simulink model "NSFsim_syn_2023"  (R2020b)
settings: Solver=FixedStepAuto  StartTime=0.0  StopTime=10  FixedStep=tstep  RelTol=1e-3
model workspace (MAT data in the model file):
  GSorder = 3
  TargetTime = 1
  blankingDur = 0.012
  mwavedur = 0.01
  rngseed = 1000
  stimfreq = 20
  tstep = 0.0001
  wc = 0.6
libraries: dspstat3 x4
settings Model: OrderedModelArguments=off  Creator=akif  LastModifiedBy=akif
settings SolverCC: AlgebraicLoopSolver=LineSearch
settings DebuggingCC: ArithmeticOperatorsInVariantConditions=warning
settings SFSimCC: CustomCodeUndefinedFunction=UseInterfaceOnly

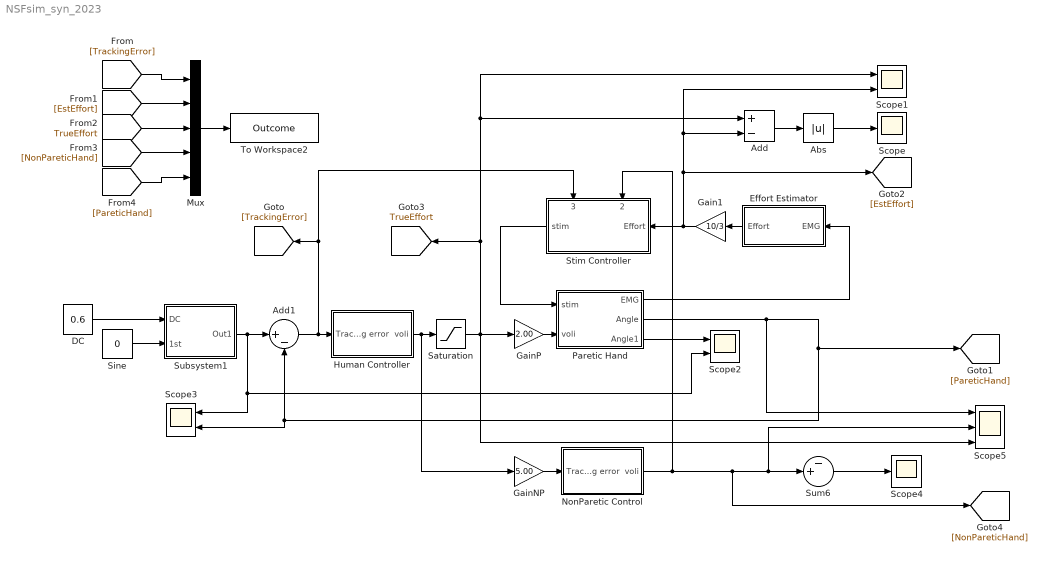
== system NSFsim_syn_2023 ==
  Abs : Abs
  Add : Sum  Inputs=+-
  Add1 : Sum  Inputs=|+-  InputSameDT=on  AccumDataTypeStr=double  OutDataTypeStr=Inherit: Inherit via back propagation
  DC : Constant  Value=0.6
  Effort Estimator : Subsystem
  Gain1 : Gain  Gain=10/3
  GainNP : Gain  Gain=5.00
  GainP : Gain  Gain=2.00
  Human Controller : Subsystem
  Mux : Mux  Inputs=5
  NonParetic Control : Subsystem
  Paretic Hand : Subsystem
  Saturation : Saturate  UpperLimit=0.3  LowerLimit=0
  Scope : Scope
  Scope1 : Scope  NumInputPorts=2
  Scope2 : Scope  NumInputPorts=2
  Scope3 : Scope  NumInputPorts=2
  Scope4 : Scope
  Scope5 : Scope  NumInputPorts=3
  Sine : Constant  Value=0
  Stim Controller : Subsystem
      settings: PortSchema="{\"entries\":[{\"content\":{\"sides\":[{\"content\":{\"connectorIds\":[\"In1\"]},\"type\":\"ConnectorPlacement.EquallySpacedRectSide\",\"uuid\":\"20982ba9-d3c9-405a-8644-0483e80e19b0\"},{\"content\":{\"connectorIds\":[\"Out1\"],\"side\":\"RIGHT\"},\"type\":\"ConnectorPlacement.EquallySpacedRectSide\",\"uuid\":\"dfaac367-100c-4435-9839-729069c8d6e0\"},{\"content\":{\"connectorIds\":[\"In2\",\"In3\"],\"side\":\"TOP\"},\"type\":\"ConnectorPlacement.EquallySpacedRectSide\",\"uuid\":\"458cbc31-cb02-49e5-bc75-9e60cc365810\"},{\"content\":{\"connectorIds\":[],\"side\":\"BOTTOM\"},\"type\":\"ConnectorPlacement.EquallySpacedRectSide\",\"uuid\":\"acd73276-1957-4a21-a6ea-49f87643696e\"}]},\"type\":\"ConnectorPlacement.EquallySpacedConnector\",\"uuid\":\"2bd25145-db49-42b2-9c0d-ce7d978301fd\"}],\"packageUris\":[\"http://schema.mathworks.com/mf0/Connector/19700101\"],\"version\":\"1.0\"}"
  Subsystem1 : Subsystem
  Sum6 : Sum  Inputs=-+|
  To Workspace2 : ToWorkspace  VariableName=Outcome  SampleTime=tstep*100
      settings: Save2DSignal=2-D array (concatenate along first dimension)
  tag scope: TrueEffort=global
  wires:
  NonParetic Control/1(voli) -> Scope5/2, Sum6/2, [NonPareticHand], Stim Controller/2(NP hand angle)
  [TrackingError] -> Mux/1
  [TrueEffort] -> Mux/3
  [EstEffort] -> Mux/2
  [NonPareticHand] -> Mux/4
  [PareticHand] -> Mux/5
  Mux/1 -> To Workspace2/1
  GainNP/1 -> NonParetic Control/1(Tracking error)
  Paretic Hand/3(Angle1) -> Scope2/1
  Stim Controller/1(stim) -> Paretic Hand/1(stim)
  Gain1/1 -> Scope1/2, Add/2, [EstEffort], Stim Controller/1(Effort)
  Add/1 -> Abs/1
  Abs/1 -> Scope/1
  Add1/1 -> Stim Controller/3(Tracking Error), [TrackingError], Human Controller/1(Tracking error)
  Subsystem1/1(Out1) -> Scope3/1, Scope2/2, Add1/1
  Sine/1 -> Subsystem1/2(1st)
  Sum6/1 -> Scope4/1
  DC/1 -> Subsystem1/1(DC)
  Paretic Hand/1(EMG) -> Effort Estimator/1(EMG)
  Paretic Hand/2(Angle) -> Scope5/1, Scope3/2, Add1/2, [PareticHand]
  Human Controller/1(voli) -> GainNP/1, Saturation/1
  GainP/1 -> Paretic Hand/2(voli)
  Saturation/1 -> Scope5/3, GainP/1, [TrueEffort], Scope1/1, Add/1
  Effort Estimator/1(Effort) -> Gain1/1

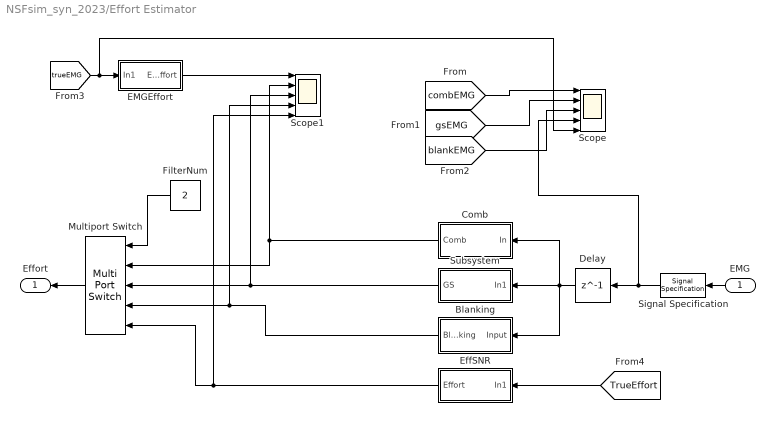
== system NSFsim_syn_2023/Effort Estimator ==
  EMG : Inport
  Blanking : Subsystem
  Comb : Subsystem
  Delay : Delay  DelayLength=1  SampleTime=tstep
  EMGEffort : Subsystem
  EffSNR : Subsystem
  FilterNum : Constant  Value=2
  Multiport Switch : MultiPortSwitch  Inputs=4
  Scope : Scope  NumInputPorts=5
  Scope1 : Scope  NumInputPorts=5
  Signal Specification : SignalSpecification  Dimensions=1
  Subsystem : Subsystem
  Effort : Outport
  wires:
  Delay/1 -> Subsystem/1(In1), Blanking/1(Input), Comb/1(In)
  EMG/1 -> Signal Specification/1
  Multiport Switch/1 -> Effort/1
  Comb/1(Comb) -> Scope1/2, Multiport Switch/2
  Subsystem/1(GS) -> Scope1/3, Multiport Switch/3
  Blanking/1(Blanking) -> Scope1/4, Multiport Switch/4
  FilterNum/1 -> Multiport Switch/1
  Signal Specification/1 -> Scope/4, Delay/1
  [combEMG] -> Scope/1
  [gsEMG] -> Scope/2
  [blankEMG] -> Scope/3
  [trueEMG] -> Scope/5, EMGEffort/1(In1)
  EMGEffort/1(EMGEffort) -> Scope1/1
  [TrueEffort] -> EffSNR/1(In1)
  EffSNR/1(Effort) -> Scope1/5, Multiport Switch/5

== system NSFsim_syn_2023/Human Controller ==
  Tracking error : Inport
  Gain : Gain  Commented=on
  Gain1 : Gain
  Integrator : Integrator  Commented=on
  Subsystem : Subsystem  Commented=on
  Transfer Fcn1 : TransferFcn  Commented=on  Numerator=[2*pi*5]  Denominator=[1 2*pi*5]
  Transfer Fcn2 : TransferFcn  Numerator=[1 2]  Denominator=[1 0 ]
  Transport Delay : TransportDelay  Commented=on  DelayTime=0.1
  Transport Delay1 : TransportDelay  DelayTime=0.1
  voli : Outport
  wires:
  Transfer Fcn2/1 -> Transport Delay1/1
  Gain1/1 -> Transfer Fcn2/1
  Gain/1 -> Integrator/1
  Integrator/1 -> Transport Delay/1
  Transport Delay1/1 -> voli/1
  Tracking error/1 -> Gain1/1

== system NSFsim_syn_2023/NonParetic Control ==
  Tracking error : Inport
  Gain : Gain
  Integrator : Integrator
  Integrator1 : Integrator
  Saturation : Saturate  UpperLimit=1  LowerLimit=0
  Subsystem : Subsystem
  Transfer Fcn : TransferFcn  Denominator=[1 2]
  Transport Delay : TransportDelay  DelayTime=0.1
  voli : Outport
  wires:
  Tracking error/1 -> Transfer Fcn/1, Gain/1
  Gain/1 -> Integrator/1
  Integrator/1 -> Transport Delay/1
  Saturation/1 -> voli/1
  Transfer Fcn/1 -> Saturation/1

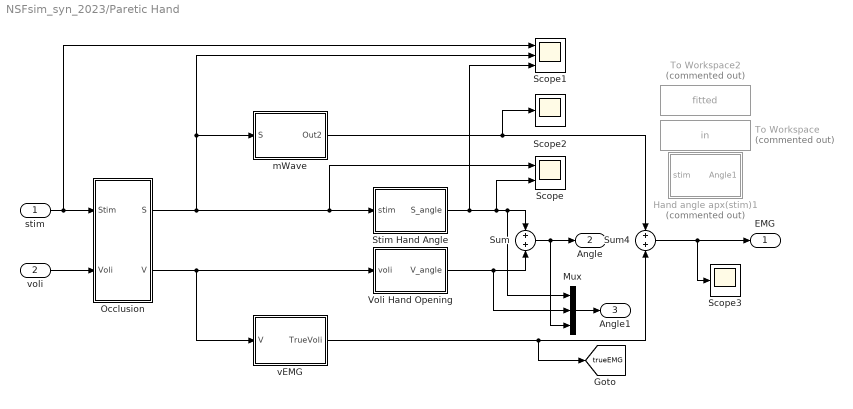
== system NSFsim_syn_2023/Paretic Hand ==
  stim : Inport
  voli : Inport  Port=2
  Hand angle apx(stim)1 : Subsystem  Commented=on
  Mux : Mux  Inputs=3
  Occlusion : Subsystem
  Scope : Scope  NumInputPorts=2
  Scope1 : Scope  NumInputPorts=3
  Scope2 : Scope
  Scope3 : Scope
  Stim Hand Angle : Subsystem
  Sum : Sum  Inputs=+|+
  Sum4 : Sum  Inputs=+|+
  To Workspace : ToWorkspace  Commented=on  VariableName=in  SampleTime=tstep*100
      settings: Save2DSignal=2-D array (concatenate along first dimension)
  To Workspace2 : ToWorkspace  Commented=on  VariableName=fitted  SampleTime=tstep*10
      settings: Save2DSignal=2-D array (concatenate along first dimension)
  Voli Hand Opening : Subsystem
  mWave : Subsystem
  vEMG : Subsystem
  EMG : Outport
  Angle : Outport  Port=2
  Angle1 : Outport  Port=3
  tag scope: trueEMG=global
  wires:
  vEMG/1(TrueVoli) -> [trueEMG], Sum4/2
  Sum4/1 -> Scope3/1, EMG/1
  Mux/1 -> Angle1/1
  mWave/1(Out2) -> Scope2/1, Sum4/1
  Sum/1 -> Mux/3, Angle/1
  Stim Hand Angle/1(S_angle) -> Scope1/3, Scope/2, Mux/1, Sum/1
  Voli Hand Opening/1(V_angle) -> Mux/2, Sum/2
  stim/1 -> Scope1/1, Occlusion/1(Stim)
  voli/1 -> Occlusion/2(Voli)
  Occlusion/1(S) -> Scope/1, Stim Hand Angle/1(stim), Scope1/2, mWave/1(S)
  Occlusion/2(V) -> vEMG/1(V), Voli Hand Opening/1(voli)

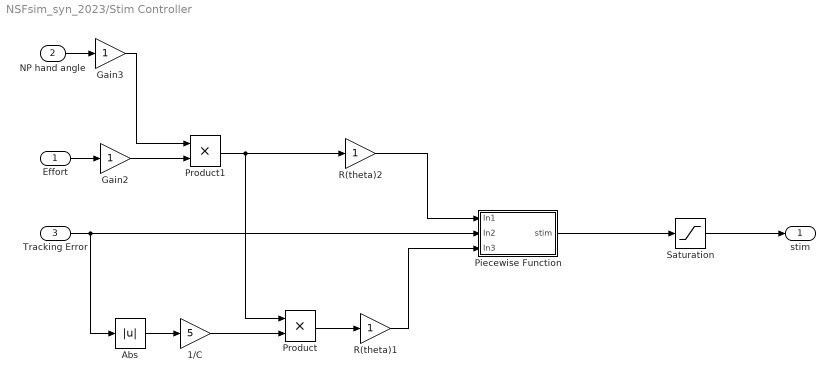
== system NSFsim_syn_2023/Stim Controller ==
  Effort : Inport
  NP hand angle : Inport  Port=2
  Tracking Error : Inport  Port=3
  1/C : Gain  Gain=5
  Abs : Abs
  Gain2 : Gain
  Gain3 : Gain
  Piecewise Function : Subsystem
  Product : Product
  Product1 : Product
  R(theta)1 : Gain
  R(theta)2 : Gain
  Saturation : Saturate  UpperLimit=1  LowerLimit=0
  stim : Outport
  wires:
  Product/1 -> R(theta)1/1
  1/C/1 -> Product/2
  R(theta)1/1 -> Piecewise Function/3(In3)
  Effort/1 -> Gain2/1
  NP hand angle/1 -> Gain3/1
  Product1/1 -> R(theta)2/1, Product/1
  Saturation/1 -> stim/1
  R(theta)2/1 -> Piecewise Function/1(In1)
  Abs/1 -> 1/C/1
  Gain2/1 -> Product1/2
  Tracking Error/1 -> Abs/1, Piecewise Function/2(In2)
  Gain3/1 -> Product1/1
  Piecewise Function/1(stim) -> Saturation/1

== system NSFsim_syn_2023/Subsystem1 ==
  DC : Inport
  1st : Inport  Port=2
  Add2 : Sum
  Product : Product  Inputs=3
  Product1 : Product
  Sine Wave : Sin  Frequency=2*pi/2  SampleTime=0
  Step : Step  Time=TargetTime  SampleTime=0
  Out1 : Outport
  wires:
  Add2/1 -> Out1/1
  Product1/1 -> Add2/1
  Product/1 -> Add2/2
  Step/1 -> Product/1, Product1/2
  DC/1 -> Product1/1
  Sine Wave/1 -> Product/3
  1st/1 -> Product/2

== system NSFsim_syn_2023/Effort Estimator/Blanking ==
  Input : Inport
  Logical Operator : Logic  Operator=NOT  AllPortsSameDT=off  OutDataTypeStr=boolean
  MAV1 : Subsystem
  Product : Product
  Pulse Generator1 : DiscretePulseGenerator  Commented=on  PulseType=Time based  Period=round(1/stimfreq,4)  PulseWidth=round(blankingDur*stimfreq,4)*100  PhaseDelay=round(1/stimfreq/2-mwavedur/2,4)
  Pulse Generator2 : DiscretePulseGenerator  Period=round(1/stimfreq/tstep)  PulseWidth=round(mwavedur/tstep)  PhaseDelay=round(1/stimfreq/tstep/2-mwavedur/tstep/2)  SampleTime=-1
  Scope : Scope
  Blanking : Outport
  tag scope: blankEMG=global
  wires:
  Input/1 -> Product/2
  Product/1 -> [blankEMG], MAV1/1(In1), Scope/1
  Logical Operator/1 -> Product/1
  MAV1/1(Effort) -> Blanking/1
  Pulse Generator2/1 -> Logical Operator/1

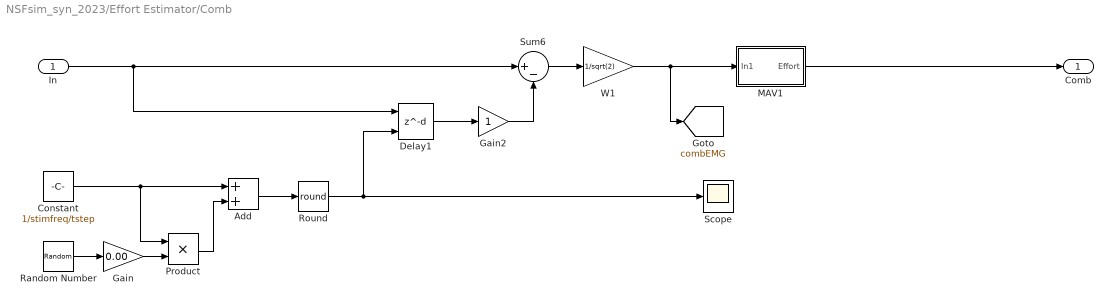
== system NSFsim_syn_2023/Effort Estimator/Comb ==
  In : Inport
  Add : Sum
  Constant : Constant  Value=1/stimfreq/tstep
  Delay1 : Delay  DelayLengthSource=Input port  DelayLength=1  DelayLengthUpperLimit=10000
      settings: InputPortMap=u0,p1
  Gain : Gain  Gain=0.00
  Gain2 : Gain
  MAV1 : Subsystem
  Product : Product
  Random Number : RandomNumber  SampleTime=round(1/stimfreq,4)
  Round : Rounding  Operator=round
  Scope : Scope
  Sum6 : Sum  Inputs=|+-
  W1 : Gain  Gain=1/sqrt(2)
  Comb : Outport
  tag scope: combEMG=global
  wires:
  Gain2/1 -> Sum6/2
  Sum6/1 -> W1/1
  In/1 -> Sum6/1, Delay1/1
  Delay1/1 -> Gain2/1
  Constant/1 -> Product/1, Add/1
  Add/1 -> Round/1
  Product/1 -> Add/2
  Round/1 -> Delay1/2, Scope/1
  Random Number/1 -> Gain/1
  Gain/1 -> Product/2
  W1/1 -> [combEMG], MAV1/1(In1)
  MAV1/1(Effort) -> Comb/1

== system NSFsim_syn_2023/Effort Estimator/EMGEffort ==
  In1 : Inport
  Abs : Abs
  Gain : Gain  Gain=5
  Moving Average : dspstat3/Moving Average  Method=Sliding window  ForgettingFactorPort=off  SpecifyWindowLength=on  WindowLength=round(1/stimfreq/tstep)  ForgettingFactor=0.9  SimulateUsing=Code generation
  ZOH : Subsystem  Commented=on
  Zero-Order Hold : ZeroOrderHold  SampleTime=round(1/stimfreq,4)
  EMGEffort : Outport
  wires:
  In1/1 -> Abs/1
  Abs/1 -> Moving Average/1
  Moving Average/1 -> Zero-Order Hold/1
  Zero-Order Hold/1 -> Gain/1
  Gain/1 -> EMGEffort/1

== system NSFsim_syn_2023/Effort Estimator/EffSNR ==
  In1 : Inport
  Abs : Abs
  Add : Sum
  Gain : Gain  Gain=1.000
  Product : Product
  Random Number : RandomNumber  SampleTime=round(1/stimfreq,4)
  Zero-Order Hold : ZeroOrderHold  SampleTime=round(1/stimfreq,4)
  Effort : Outport
  wires:
  In1/1 -> Add/2, Product/2
  Product/1 -> Add/1
  Gain/1 -> Product/1
  Zero-Order Hold/1 -> Effort/1
  Random Number/1 -> Gain/1
  Abs/1 -> Zero-Order Hold/1
  Add/1 -> Abs/1

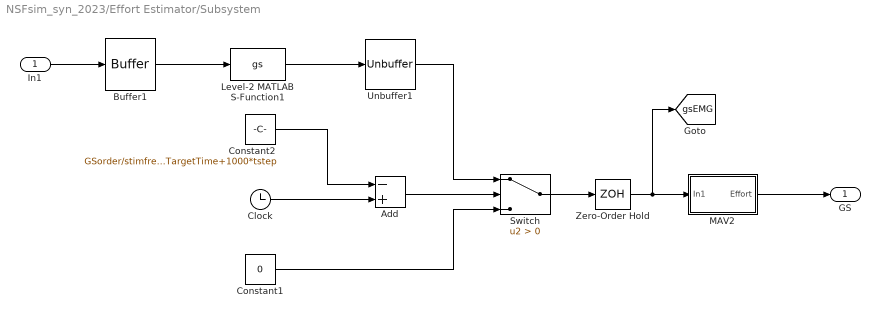
== system NSFsim_syn_2023/Effort Estimator/Subsystem ==
  In1 : Inport
  Add : Sum  Inputs=-+
  Buffer1 : Buffer  N=round(1/stimfreq/tstep)  OutputFrames=off
  Clock : Clock
  Constant1 : Constant  Value=0
  Constant2 : Constant  Value=GSorder/stimfreq+TargetTime+1000*tstep
  Level-2 MATLAB S-Function1 : M-S-Function  FunctionName=gs  Parameters=GSorder,round(1/stimfreq/tstep),tstep,stimfreq
  MAV2 : Subsystem
  Switch : Switch  Criteria=u2 > Threshold
  Unbuffer1 : Unbuffer
  Zero-Order Hold : ZeroOrderHold  SampleTime=-1
  GS : Outport
  tag scope: gsEMG=global
  wires:
  In1/1 -> Buffer1/1
  Constant2/1 -> Add/1
  Level-2 MATLAB S-Function1/1 -> Unbuffer1/1
  Add/1 -> Switch/2
  Unbuffer1/1 -> Switch/1
  Buffer1/1 -> Level-2 MATLAB S-Function1/1
  Constant1/1 -> Switch/3
  Zero-Order Hold/1 -> [gsEMG], MAV2/1(In1)
  Clock/1 -> Add/2
  Switch/1 -> Zero-Order Hold/1
  MAV2/1(Effort) -> GS/1

== system NSFsim_syn_2023/Human Controller/Subsystem ==
  note: here used as saturation
  note: maps input to nonliear static eqn
  note: input between 0 1
  In1 : Inport
  Constant : Constant  Value=-5
  Fcn : Fcn  Expr=exp(u(1))/(1+exp(u(1)))
  Gain1 : Gain  Gain=10
  Scope : Scope  NumInputPorts=2
  Sum : Sum  Inputs=|++
  Out1 : Outport
  wires:
  In1/1 -> Gain1/1, Scope/2
  Sum/1 -> Fcn/1
  Gain1/1 -> Sum/1
  Constant/1 -> Sum/2
  Fcn/1 -> Out1/1, Scope/1

== system NSFsim_syn_2023/NonParetic Control/Subsystem ==
  note: here used as saturation
  note: maps input to nonliear static eqn
  note: input between 0 1
  In1 : Inport
  Constant : Constant  Value=-5
  Fcn : Fcn  Expr=exp(u(1))/(1+exp(u(1)))
  Gain1 : Gain  Gain=10
  Scope : Scope  NumInputPorts=2
  Sum : Sum  Inputs=|++
  Out1 : Outport
  wires:
  In1/1 -> Gain1/1, Scope/2
  Sum/1 -> Fcn/1
  Gain1/1 -> Sum/1
  Constant/1 -> Sum/2
  Fcn/1 -> Out1/1, Scope/1

== system NSFsim_syn_2023/Paretic Hand/Hand angle apx(stim)1 ==
  stim : Inport
  Gain3 : Gain
  Subsystem : Subsystem
  Transfer Fcn : TransferFcn  Denominator=[.2 1]
  Angle1 : Outport
  wires:
  stim/1 -> Transfer Fcn/1
  Transfer Fcn/1 -> Gain3/1
  Gain3/1 -> Angle1/1

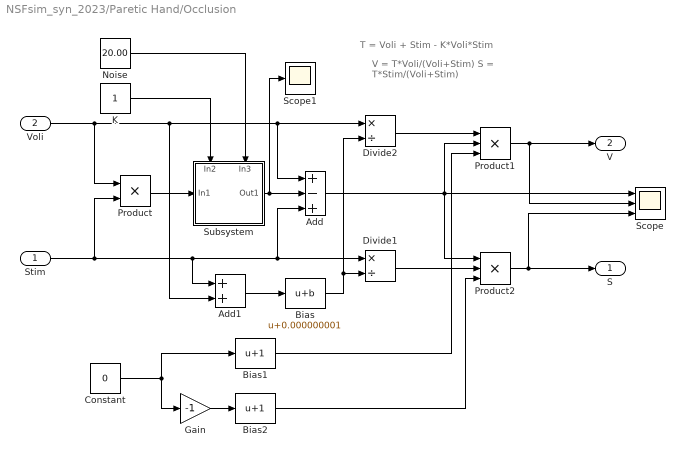
== system NSFsim_syn_2023/Paretic Hand/Occlusion ==
  note: V = T*Voli/(Voli+Stim)
      | S = T*Stim/(Voli+Stim)
  note: T = Voli + Stim - K*Voli*Stim
  Stim : Inport
  Voli : Inport  Port=2
  Add : Sum  Inputs=+-+
  Add1 : Sum
  Bias : Bias  Bias=0.000000001
  Bias1 : Bias  Bias=1
  Bias2 : Bias  Bias=1
  Constant : Constant  Value=0
  Divide1 : Product  Inputs=*/
  Divide2 : Product  Inputs=*/
  Gain : Gain  Gain=-1
  K : Constant
  Noise : Constant  Value=20.00
  Product : Product
  Product1 : Product  Inputs=3
  Product2 : Product  Inputs=3
  Scope : Scope  NumInputPorts=3
  Scope1 : Scope
  Subsystem : Subsystem
      settings: PortSchema="{\"entries\":[{\"content\":{\"sides\":[{\"content\":{\"connectorIds\":[\"In1\"]},\"type\":\"ConnectorPlacement.EquallySpacedRectSide\",\"uuid\":\"4ccf8a84-1781-40d8-90f2-eda5d680272e\"},{\"content\":{\"connectorIds\":[\"Out1\"],\"side\":\"RIGHT\"},\"type\":\"ConnectorPlacement.EquallySpacedRectSide\",\"uuid\":\"e5fa6e2b-5207-422b-9a6d-ff33f0c06180\"},{\"content\":{\"connectorIds\":[\"In2\",\"In3\"],\"side\":\"TOP\"},\"type\":\"ConnectorPlacement.EquallySpacedRectSide\",\"uuid\":\"eb5b22a9-1bab-4754-aed5-081055618c5e\"},{\"content\":{\"connectorIds\":[],\"side\":\"HIDDEN\"},\"type\":\"ConnectorPlacement.EquallySpacedRectSide\",\"uuid\":\"29a39b3b-31d7-430f-b6b0-cf2df9335134\"}]},\"type\":\"ConnectorPlacement.EquallySpacedConnector\",\"uuid\":\"308de845-bfcc-4591-8d67-89c6c737dd83\"}],\"packageUris\":[\"http://schema.mathworks.com/mf0/Connector/R2020b\"],\"version\":\"1.0\"}"
  S : Outport
  V : Outport  Port=2
  wires:
  Voli/1 -> Product/1, Divide2/1, Add/1, Add1/2
  Add/1 -> Product1/2, Product2/1, Scope/1
  Product/1 -> Subsystem/1(In1)
  Subsystem/1(Out1) -> Add/2, Scope1/1
  Divide1/1 -> Product2/2
  Divide2/1 -> Product1/1
  Product1/1 -> V/1, Scope/2
  Product2/1 -> Scope/3, S/1
  K/1 -> Subsystem/2(In2)
  Noise/1 -> Subsystem/3(In3)
  Stim/1 -> Add1/1, Add/3, Divide1/1, Product/2
  Add1/1 -> Bias/1
  Bias/1 -> Divide2/2, Divide1/2
  Bias1/1 -> Product1/3
  Constant/1 -> Bias1/1, Gain/1
  Bias2/1 -> Product2/3
  Gain/1 -> Bias2/1

== system NSFsim_syn_2023/Paretic Hand/Stim Hand Angle ==
  stim : Inport
  Gain3 : Gain
  Subsystem : Subsystem
  Transfer Fcn : TransferFcn  Denominator=[0.300 1]
  S_angle : Outport
  wires:
  Gain3/1 -> S_angle/1
  Transfer Fcn/1 -> Gain3/1
  stim/1 -> Transfer Fcn/1

== system NSFsim_syn_2023/Paretic Hand/Voli Hand Opening ==
  voli : Inport
  Gain3 : Gain
  Subsystem : Subsystem
  Transfer Fcn : TransferFcn  Denominator=[1 3]
  V_angle : Outport
  wires:
  Transfer Fcn/1 -> Gain3/1
  Gain3/1 -> V_angle/1
  voli/1 -> Transfer Fcn/1

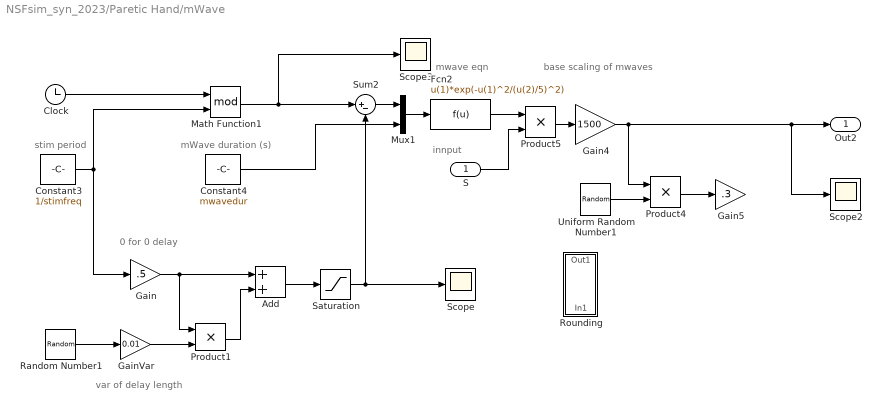
== system NSFsim_syn_2023/Paretic Hand/mWave ==
  note: 0 for 0 delay
  note: innput
  note: var of delay length
  note: stim period
  note: mWave duration (s)
  note: mwave eqn
  note: base scaling of mwaves
  S : Inport
  Add : Sum
  Clock : Clock
  Constant3 : Constant  Value=1/stimfreq
  Constant4 : Constant  Value=mwavedur  VectorParams1D=off
  Fcn2 : Fcn  Expr=u(1)*exp(-u(1)^2/(u(2)/5)^2)
  Gain : Gain  Gain=.5
  Gain4 : Gain  Gain=1500
  Gain5 : Gain  Gain=.3
  GainVar : Gain  Gain=0.01
  Math Function1 : Math  Operator=mod  SaturateOnIntegerOverflow=on
  Mux1 : Mux  Inputs=2
  Product1 : Product
  Product4 : Product
  Product5 : Product
  Random Number1 : RandomNumber  Seed=rngseed*12  SampleTime=round(1/stimfreq,4)
  Rounding : Subsystem
  Saturation : Saturate  UpperLimit=1/stimfreq-1/stimfreq/10  LowerLimit=1/stimfreq/10
  Scope : Scope
  Scope2 : Scope
  Scope3 : Scope
  Sum2 : Sum  Inputs=|+-
  Uniform Random Number1 : UniformRandomNumber  Seed=1234  SampleTime=tstep
  Out2 : Outport  VectorParamsAs1DForOutWhenUnconnected=off
  wires:
  S/1 -> Product5/2
  Constant3/1 -> Math Function1/2, Gain/1
  Constant4/1 -> Mux1/2
  Sum2/1 -> Mux1/1
  Math Function1/1 -> Scope3/1, Sum2/1
  Mux1/1 -> Fcn2/1
  Product4/1 -> Gain5/1
  Uniform Random Number1/1 -> Product4/2
  Gain4/1 -> Out2/1, Scope2/1, Product4/1
  Fcn2/1 -> Product5/1
  Product5/1 -> Gain4/1
  Clock/1 -> Math Function1/1
  Random Number1/1 -> GainVar/1
  Gain/1 -> Product1/1, Add/1
  GainVar/1 -> Product1/2
  Product1/1 -> Add/2
  Add/1 -> Saturation/1
  Saturation/1 -> Sum2/2, Scope/1

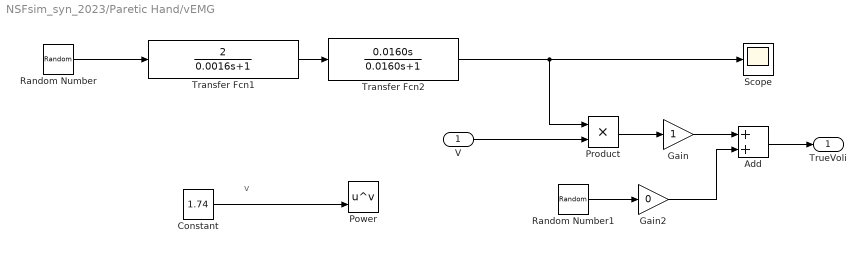
== system NSFsim_syn_2023/Paretic Hand/vEMG ==
  note: v
  V : Inport
  Add : Sum
  Constant : Constant  Value=1.74
  Gain : Gain
  Gain2 : Gain  Gain=0
  Power : Math  Operator=pow  SignedPower=on  SaturateOnIntegerOverflow=on
  Product : Product
  Random Number : RandomNumber  Seed=rngseed*1.2
  Random Number1 : RandomNumber  Seed=4445
  Scope : Scope
  Transfer Fcn1 : TransferFcn  Numerator=[2]  Denominator=[0.0016 1]
  Transfer Fcn2 : TransferFcn  Numerator=[0.0160 0]  Denominator=[0.0160 1]
  TrueVoli : Outport
  wires:
  V/1 -> Product/2
  Constant/1 -> Power/2
  Random Number/1 -> Transfer Fcn1/1
  Transfer Fcn1/1 -> Transfer Fcn2/1
  Product/1 -> Gain/1
  Transfer Fcn2/1 -> Scope/1, Product/1
  Gain/1 -> Add/1
  Add/1 -> TrueVoli/1
  Random Number1/1 -> Gain2/1
  Gain2/1 -> Add/2

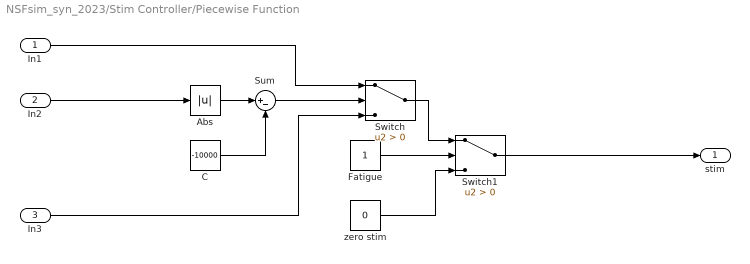
== system NSFsim_syn_2023/Stim Controller/Piecewise Function ==
  In1 : Inport
  In2 : Inport  Port=2
  In3 : Inport  Port=3
  Abs : Abs
  C : Constant  Value=-10000
  Fatigue : Constant
  Sum : Sum  Inputs=|+-
  Switch : Switch  Criteria=u2 > Threshold
  Switch1 : Switch  Criteria=u2 > Threshold
  zero stim : Constant  Value=0
  stim : Outport
  wires:
  Abs/1 -> Sum/1
  Fatigue/1 -> Switch1/2
  In3/1 -> Switch/3
  Switch/1 -> Switch1/1
  In1/1 -> Switch/1
  zero stim/1 -> Switch1/3
  In2/1 -> Abs/1
  C/1 -> Sum/2
  Sum/1 -> Switch/2
  Switch1/1 -> stim/1

== system NSFsim_syn_2023/Effort Estimator/Blanking/MAV1 ==
  In1 : Inport
  Abs : Abs
  BlankingGain : Gain  Gain=5  OutDataTypeStr=Inherit: Same as input
  Moving Average : dspstat3/Moving Average  Method=Sliding window  ForgettingFactorPort=off  SpecifyWindowLength=on  WindowLength=round(1/stimfreq/tstep)  ForgettingFactor=0.9  SimulateUsing=Code generation
  Scope : Scope  NumInputPorts=3
  ZOH : Subsystem  Commented=on
  Zero-Order Hold : ZeroOrderHold  SampleTime=round(1/stimfreq,4)
  Effort : Outport
  wires:
  In1/1 -> Abs/1
  Abs/1 -> Scope/3, Moving Average/1
  Moving Average/1 -> Scope/1, Zero-Order Hold/1
  Zero-Order Hold/1 -> Scope/2, BlankingGain/1
  BlankingGain/1 -> Effort/1

== system NSFsim_syn_2023/Effort Estimator/Comb/MAV1 ==
  In1 : Inport
  Abs : Abs
  CombGain : Gain  Gain=5  OutDataTypeStr=Inherit: Same as input
  Moving Average : dspstat3/Moving Average  Method=Sliding window  ForgettingFactorPort=off  SpecifyWindowLength=on  WindowLength=round(1/stimfreq/tstep)  ForgettingFactor=0.9  SimulateUsing=Code generation
  ZOH : Subsystem  Commented=on
  Zero-Order Hold : ZeroOrderHold  SampleTime=round(1/stimfreq,4)
  Effort : Outport
  wires:
  In1/1 -> Abs/1
  Abs/1 -> Moving Average/1
  Moving Average/1 -> Zero-Order Hold/1
  Zero-Order Hold/1 -> CombGain/1
  CombGain/1 -> Effort/1

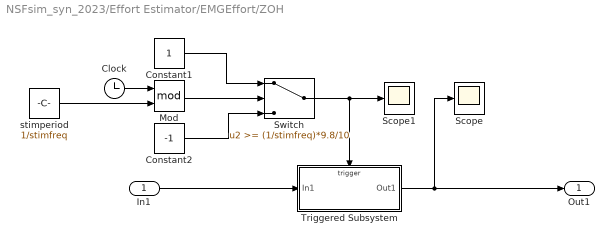
== system NSFsim_syn_2023/Effort Estimator/EMGEffort/ZOH ==
  In1 : Inport
  Clock : Clock
  Constant1 : Constant
  Constant2 : Constant  Value=-1
  Mod : Math  Operator=mod  SaturateOnIntegerOverflow=on
  Scope : Scope
  Scope1 : Scope
  Switch : Switch  Threshold=(1/stimfreq)*9.8/10
  Triggered Subsystem : Subsystem  TreatAsAtomicUnit=on
  stimperiod : Constant  Value=1/stimfreq
  Out1 : Outport
  wires:
  Switch/1 -> Triggered Subsystem/Trigger, Scope1/1
  In1/1 -> Triggered Subsystem/1(In1)
  Constant1/1 -> Switch/1
  Mod/1 -> Switch/2
  Constant2/1 -> Switch/3
  stimperiod/1 -> Mod/2
  Clock/1 -> Mod/1
  Triggered Subsystem/1(Out1) -> Out1/1, Scope/1

== system NSFsim_syn_2023/Effort Estimator/Subsystem/MAV2 ==
  In1 : Inport
  Abs : Abs
  GSGain : Gain  Gain=8  OutDataTypeStr=Inherit: Same as input
  Moving Average : dspstat3/Moving Average  Method=Sliding window  ForgettingFactorPort=off  SpecifyWindowLength=on  WindowLength=round(1/stimfreq/tstep)  ForgettingFactor=0.9  SimulateUsing=Code generation
  ZOH : Subsystem  Commented=on
  Zero-Order Hold : ZeroOrderHold  SampleTime=round(1/stimfreq,4)
  Effort : Outport
  wires:
  In1/1 -> Abs/1
  Abs/1 -> Moving Average/1
  Moving Average/1 -> Zero-Order Hold/1
  Zero-Order Hold/1 -> GSGain/1
  GSGain/1 -> Effort/1

== system NSFsim_syn_2023/Paretic Hand/Hand angle apx(stim)1/Subsystem ==
  note: input between 0 1
  note: maps input to nonliear static eqn
  In1 : Inport
  Constant : Constant  Value=-5
  Fcn : Fcn  Expr=exp(u(1))/(1+exp(u(1)))
  Gain1 : Gain  Gain=10
  Scope : Scope  NumInputPorts=2
  Sum : Sum  Inputs=|++
  Out1 : Outport
  wires:
  Fcn/1 -> Scope/1, Out1/1
  Constant/1 -> Sum/2
  Gain1/1 -> Sum/1
  Sum/1 -> Fcn/1
  In1/1 -> Scope/2, Gain1/1

== system NSFsim_syn_2023/Paretic Hand/Occlusion/Subsystem ==
  note: K
  In1 : Inport
  In2 : Inport  Port=2
  In3 : Inport  Port=3
  Add2 : Sum
  Gain : Gain  Gain=0.01
  Product5 : Product  Inputs=3
  Product6 : Product
  Random Number1 : RandomNumber  Seed=rngseed*2
  Out1 : Outport
  wires:
  In2/1 -> Product5/3, Add2/2
  Product5/1 -> Add2/1
  Add2/1 -> Product6/1
  In1/1 -> Product6/2
  Product6/1 -> Out1/1
  Gain/1 -> Product5/1
  In3/1 -> Gain/1
  Random Number1/1 -> Product5/2

== system NSFsim_syn_2023/Paretic Hand/Stim Hand Angle/Subsystem ==
  note: maps input to nonliear static eqn
  note: input between 0 1
  In1 : Inport
  Constant : Constant  Value=-5
  Fcn : Fcn  Expr=exp(u(1))/(1+exp(u(1)))
  Gain1 : Gain  Gain=10
  Scope : Scope  NumInputPorts=2
  Sum : Sum  Inputs=|++
  Out1 : Outport
  wires:
  In1/1 -> Gain1/1, Scope/2
  Sum/1 -> Fcn/1
  Gain1/1 -> Sum/1
  Constant/1 -> Sum/2
  Fcn/1 -> Out1/1, Scope/1

== system NSFsim_syn_2023/Paretic Hand/Voli Hand Opening/Subsystem ==
  note: maps input to nonliear static eqn
  note: input between 0 1
  In1 : Inport
  Constant : Constant  Value=-5
  Fcn : Fcn  Expr=exp(u(1))/(1+exp(u(1)))
  Gain1 : Gain  Gain=10
  Gain2 : Gain  Gain=.2
  Sum : Sum  Inputs=|++
  Out1 : Outport
  wires:
  In1/1 -> Gain1/1
  Sum/1 -> Fcn/1
  Gain1/1 -> Sum/1
  Constant/1 -> Sum/2
  Fcn/1 -> Gain2/1
  Gain2/1 -> Out1/1

== system NSFsim_syn_2023/Paretic Hand/mWave/Rounding ==
  In1 : Inport
  Gain1 : Gain  Gain=tstep
  Gain2 : Gain  Gain=1/tstep
  Round : Rounding  Operator=round
  Scope : Scope  NumInputPorts=2
  Out1 : Outport
  wires:
  In1/1 -> Scope/2, Gain2/1
  Gain1/1 -> Scope/1, Out1/1
  Round/1 -> Gain1/1
  Gain2/1 -> Round/1

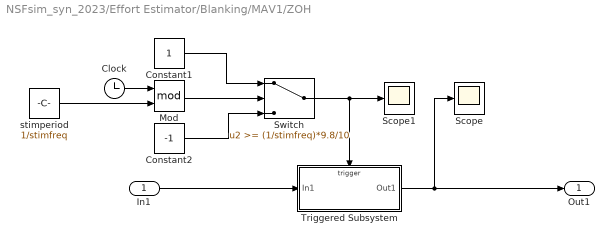
== system NSFsim_syn_2023/Effort Estimator/Blanking/MAV1/ZOH ==
  In1 : Inport
  Clock : Clock
  Constant1 : Constant
  Constant2 : Constant  Value=-1
  Mod : Math  Operator=mod  SaturateOnIntegerOverflow=on
  Scope : Scope
  Scope1 : Scope
  Switch : Switch  Threshold=(1/stimfreq)*9.8/10
  Triggered Subsystem : Subsystem  TreatAsAtomicUnit=on
  stimperiod : Constant  Value=1/stimfreq
  Out1 : Outport
  wires:
  Switch/1 -> Triggered Subsystem/Trigger, Scope1/1
  In1/1 -> Triggered Subsystem/1(In1)
  Constant1/1 -> Switch/1
  Mod/1 -> Switch/2
  Constant2/1 -> Switch/3
  stimperiod/1 -> Mod/2
  Clock/1 -> Mod/1
  Triggered Subsystem/1(Out1) -> Out1/1, Scope/1

== system NSFsim_syn_2023/Effort Estimator/Comb/MAV1/ZOH ==
  In1 : Inport
  Clock : Clock
  Constant1 : Constant
  Constant2 : Constant  Value=-1
  Mod : Math  Operator=mod  SaturateOnIntegerOverflow=on
  Scope : Scope
  Scope1 : Scope
  Switch : Switch  Threshold=(1/stimfreq)*9.8/10
  Triggered Subsystem : Subsystem  TreatAsAtomicUnit=on
  stimperiod : Constant  Value=1/stimfreq
  Out1 : Outport
  wires:
  Switch/1 -> Triggered Subsystem/Trigger, Scope1/1
  In1/1 -> Triggered Subsystem/1(In1)
  Constant1/1 -> Switch/1
  Mod/1 -> Switch/2
  Constant2/1 -> Switch/3
  stimperiod/1 -> Mod/2
  Clock/1 -> Mod/1
  Triggered Subsystem/1(Out1) -> Out1/1, Scope/1

== system NSFsim_syn_2023/Effort Estimator/EMGEffort/ZOH/Triggered Subsystem ==
  In1 : Inport
  Trigger : TriggerPort  VariantControl=Variant
  Out1 : Outport
  wires:
  In1/1 -> Out1/1

== system NSFsim_syn_2023/Effort Estimator/Subsystem/MAV2/ZOH ==
  In1 : Inport
  Clock : Clock
  Constant1 : Constant
  Constant2 : Constant  Value=-1
  Mod : Math  Operator=mod  SaturateOnIntegerOverflow=on
  Scope : Scope
  Scope1 : Scope
  Switch : Switch  Threshold=(1/stimfreq)*9.8/10
  Triggered Subsystem : Subsystem  TreatAsAtomicUnit=on
  stimperiod : Constant  Value=1/stimfreq
  Out1 : Outport
  wires:
  Switch/1 -> Triggered Subsystem/Trigger, Scope1/1
  In1/1 -> Triggered Subsystem/1(In1)
  Constant1/1 -> Switch/1
  Mod/1 -> Switch/2
  Constant2/1 -> Switch/3
  stimperiod/1 -> Mod/2
  Clock/1 -> Mod/1
  Triggered Subsystem/1(Out1) -> Out1/1, Scope/1

== system NSFsim_syn_2023/Effort Estimator/Blanking/MAV1/ZOH/Triggered Subsystem ==
  In1 : Inport
  Trigger : TriggerPort  VariantControl=Variant
  Out1 : Outport
  wires:
  In1/1 -> Out1/1

== system NSFsim_syn_2023/Effort Estimator/Comb/MAV1/ZOH/Triggered Subsystem ==
  In1 : Inport
  Trigger : TriggerPort  VariantControl=Variant
  Out1 : Outport
  wires:
  In1/1 -> Out1/1

== system NSFsim_syn_2023/Effort Estimator/Subsystem/MAV2/ZOH/Triggered Subsystem ==
  In1 : Inport
  Trigger : TriggerPort  VariantControl=Variant
  Out1 : Outport
  wires:
  In1/1 -> Out1/1
